simulink model "Lab03"  (R2023b)
settings: Solver=VariableStepAuto  StartTime=0.0  StopTime=1800  RelTol=1e-3
values from neighbouring files (symbols this model uses):
  A = [0 -1 5; 0 0 3; 0 0 -2]    [Lab01.m]    (also in Lab03.m = double(subs(A,x,x_eq)); Lab04.m = double(subs(A,[x u],[x_eq u_eq])); Lab05.m = [0 1; -3 -4])
  B = [1 1 1]'    [Lab01.m]    (also in Lab03.m = double(subs(B,u,u_eq)); Lab04.m = double(subs(B,[x u],[x_eq u_eq])); Lab05.m = [0 ; 1])
  gamma_eq = 0    [Lab03.m]
  Gb = 81    [Lab03.m]
  Ib = 15    [Lab03.m]
  n = 5/54    (= 0.0925925925926)    [Lab03.m]
  p1 = 0.003    [Lab03.m]
  p2 = 0.025    [Lab03.m]
  p3 = 0.000013    (= 1.3e-05)    [Lab03.m]
  r_eq = 16.66667    [Lab03.m]
  V1 = 12    [Lab03.m]
  VG = 126    [Lab03.m]
libraries: simulink x4
settings Model: Creator=matteo  LastModifiedBy=matteo

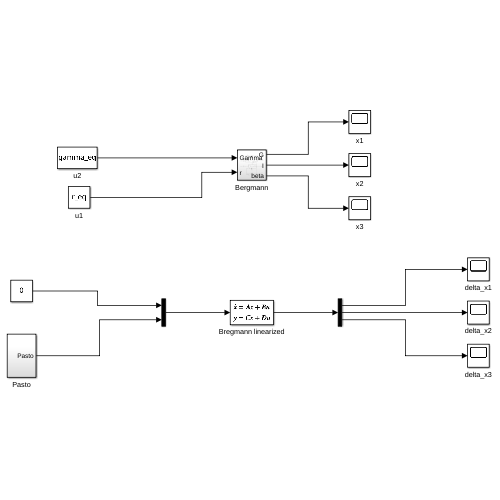
[thumbnail: Simulink's stored preview of the top-level diagram]
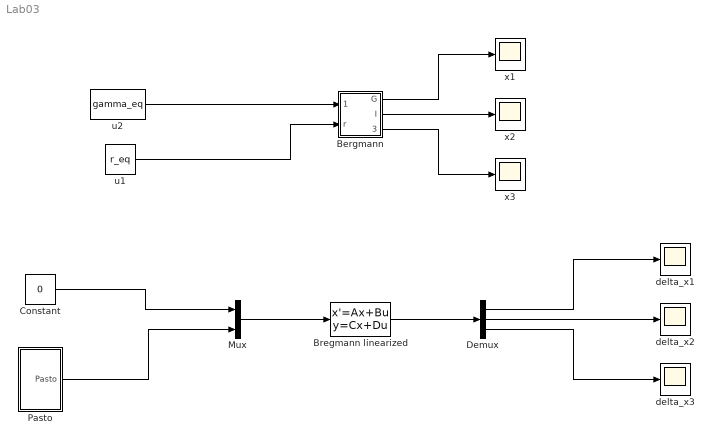
== system Lab03 ==
  Bergmann : Subsystem
  Bregmann linearized : StateSpace  A=A  B=B  C=eye(3,3)  D=zeros(3,2)  InitialCondition=[9 0 0]
  Constant : Constant  Value=0
  Demux : Demux  Outputs=3
  Mux : Mux  Inputs=2
  Pasto : Subsystem
  delta_x1 : Scope
  delta_x2 : Scope
  delta_x3 : Scope
  u1 : Constant  Value=r_eq
  u2 : Constant  Value=gamma_eq
  x1 : Scope
  x2 : Scope
  x3 : Scope
  wires:
  Bergmann/1(G) -> x1/1
  u2/1 -> Bergmann/1(Gamma)
  u1/1 -> Bergmann/2(r)
  Bergmann/2(I) -> x2/1
  Bergmann/3(beta) -> x3/1
  Bregmann linearized/1 -> Demux/1
  Mux/1 -> Bregmann linearized/1
  Demux/1 -> delta_x1/1
  Demux/2 -> delta_x2/1
  Demux/3 -> delta_x3/1
  Pasto/1(Pasto) -> Mux/2
  Constant/1 -> Mux/1

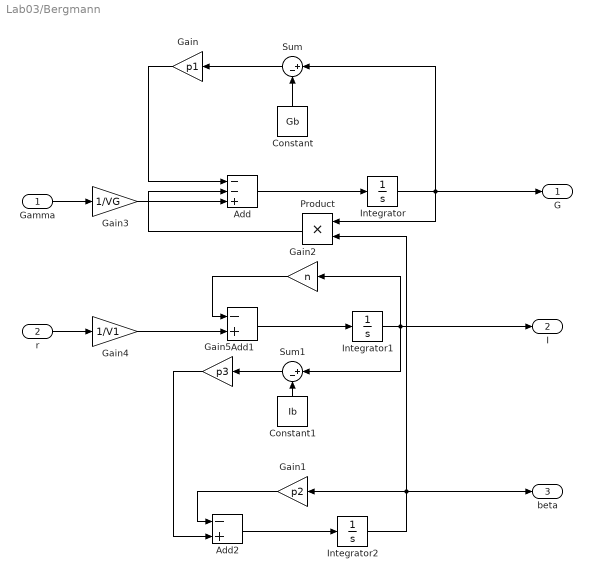
== system Lab03/Bergmann ==
  Gamma : Inport
  r : Inport  Port=2
  Add : Sum  Inputs=--+
  Add1 : Sum  Inputs=-+
  Add2 : Sum  Inputs=-+
  Constant : Constant  Value=Gb
  Constant1 : Constant  Value=Ib
  Gain : Gain  Gain=p1
  Gain1 : Gain  Gain=p2
  Gain2 : Gain  Gain=n
  Gain3 : Gain  Gain=1/VG
  Gain4 : Gain  Gain=1/V1
  Gain5 : Gain  Gain=p3
  Integrator : Integrator
  Integrator1 : Integrator
  Integrator2 : Integrator
  Product : Product
  Sum : Sum  Inputs=|+-
  Sum1 : Sum  Inputs=|+-
  G : Outport
  I : Outport  Port=2
  beta : Outport  Port=3
  wires:
  Gain4/1 -> Add1/2
  Gain3/1 -> Add/3
  Gamma/1 -> Gain3/1
  Add1/1 -> Integrator1/1
  Add2/1 -> Integrator2/1
  Constant/1 -> Sum/2
  Integrator2/1 -> Product/2, beta/1, Gain1/1
  Gain5/1 -> Add2/2
  Constant1/1 -> Sum1/2
  Gain2/1 -> Add1/1
  Integrator1/1 -> I/1, Sum1/1, Gain2/1
  Gain1/1 -> Add2/1
  Gain/1 -> Add/1
  Sum/1 -> Gain/1
  Integrator/1 -> G/1, Sum/1, Product/1
  Add/1 -> Integrator/1
  r/1 -> Gain4/1
  Sum1/1 -> Gain5/1
  Product/1 -> Add/2

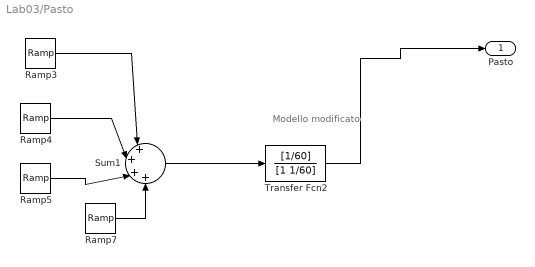
== system Lab03/Pasto ==
  note: Modello
      | modificato
  Ramp3 : simulink/Sources/Ramp  slope=12  start=0  InitialOutput=0
  Ramp4 : simulink/Sources/Ramp  slope=-12  start=30  InitialOutput=0
  Ramp5 : simulink/Sources/Ramp  slope=-12  start=90  InitialOutput=0
  Ramp7 : simulink/Sources/Ramp  slope=12  start=120  InitialOutput=0
  Sum1 : Sum  Inputs=|+|+|+|+  InputSameDT=on  SaturateOnIntegerOverflow=on  OutDataTypeStr=Inherit: Same as first input
  Transfer Fcn2 : TransferFcn  Numerator=[1/60]  Denominator=[1 1/60]
  Pasto : Outport
  wires:
  Ramp3/1 -> Sum1/1
  Ramp4/1 -> Sum1/2
  Ramp5/1 -> Sum1/3
  Ramp7/1 -> Sum1/4
  Sum1/1 -> Transfer Fcn2/1
  Transfer Fcn2/1 -> Pasto/1
